simulink model "sampleModel27"  (R2021a)
settings: Solver=VariableStepAuto  StartTime=0.0  StopTime=10.0  RelTol=1e-3
undefined symbols (not defined in the file): DiscIntNeverNeededParam, magnitude, Newton, Raphson
libraries: simulink x49, pid_lib x7
(part 2 of 2)

== system sampleModel27/cfblk83/cfblk13/cfblk7 ==
  cfblk1 : Inport
  cfblk13 : Inport  Port=2
  cfblk10 : Constant  Value=[544016772.040966]  SampleTime=1
  cfblk11 : Constant  Value=[-953538141.984181]  SampleTime=1
  cfblk12 : Subsystem
  cfblk14 : Delay  SampleTime=1
  cfblk15 : Delay  SampleTime=1
  cfblk3 : simulink/Discrete/Transfer Fcn First Order  PoleZ=0.95  ICPrevOutput=0.0  DoSatur=off
  cfblk4 : DiscreteZeroPole  Poles=[0 0.5]  Gain=1
  cfblk5 : Sum  Inputs=|++
  cfblk6 : ComplexToMagnitudeAngle
  cfblk7 : Sum  Inputs=+
  cfblk8 : Polyval  Coefs=[ +2.081618890e-019, -1.441693666e-014, +4.719686976e-010, -8.536869453e-006, +1.621573104e-001, -8.087801117e+001 ]
  cfblk9 : UnaryMinus
  cfblk2 : Outport
  wires:
  cfblk6/1 -> cfblk8/1
  cfblk1/1 -> cfblk7/1
  cfblk13/1 -> cfblk6/1
  cfblk7/1 -> cfblk5/1
  cfblk10/1 -> cfblk2/1
  cfblk6/2 -> cfblk5/2
  cfblk8/1 -> cfblk4/1
  cfblk11/1 -> cfblk12/2(cfblk13)
  cfblk5/1 -> cfblk12/3(cfblk14)
  cfblk4/1 -> cfblk12/4(cfblk15)
  cfblk12/1(cfblk2) -> cfblk9/1
  cfblk12/2(cfblk17) -> cfblk3/1
  cfblk9/1 -> cfblk14/1
  cfblk14/1 -> cfblk12/5(cfblk16)
  cfblk3/1 -> cfblk15/1
  cfblk15/1 -> cfblk12/1(cfblk1)

== system sampleModel27/cfblk83/cfblk15/cfblk14 ==
  cfblk1 : Inport
  cfblk11 : Subsystem  TreatAsAtomicUnit=on
  cfblk12 : Subsystem  TreatAsAtomicUnit=on
  cfblk13 : Subsystem  TreatAsAtomicUnit=on
  cfblk14 : Subsystem  TreatAsAtomicUnit=on
  cfblk15 : Delay
  cfblk16 : Delay
  cfblk17 : Delay
  cfblk3 : UnitDelay  SampleTime=-1  HasFrameUpgradeWarning=on
  cfblk4 : Rounding
  cfblk5 : Constant  Value=[-440599559.077869]  SampleTime=1
  cfblk6 : Constant  Value=[542136050.953861]  SampleTime=1
  cfblk7 : Constant  Value=[-811490102.664521]  SampleTime=1
  cfblk8 : If  IfExpression=u1 >= 0  SampleTime=1
  cfblk9 : If  IfExpression=u1 >= 0  SampleTime=1
  cfblk2 : Outport
  cfblk10 : Outport  Port=2
  wires:
  cfblk1/1 -> cfblk14/1(cfblk1)
  cfblk6/1 -> cfblk2/1, cfblk8/1
  cfblk14/1(cfblk2) -> cfblk4/1, cfblk11/4(cfblk16), cfblk11/5(cfblk17), cfblk12/6(cfblk15)
  cfblk12/1(cfblk2) -> cfblk10/1
  cfblk5/1 -> cfblk3/1, cfblk12/3(cfblk12), cfblk12/5(cfblk14)
  cfblk7/1 -> cfblk14/2(cfblk16)
  cfblk4/1 -> cfblk11/3(cfblk15), cfblk15/1
  cfblk3/1 -> cfblk13/3(cfblk9), cfblk12/2(cfblk11), cfblk13/4(cfblk10), cfblk12/4(cfblk13)
  cfblk13/2(cfblk11) -> cfblk12/1(cfblk1)
  cfblk12/2(cfblk16) -> cfblk11/1(cfblk1)
  cfblk12/3(cfblk17) -> cfblk11/2(cfblk14)
  cfblk8/1 -> cfblk11/Action
  cfblk8/2 -> cfblk12/Action
  cfblk9/1 -> cfblk13/Action
  cfblk9/2 -> cfblk14/Action
  cfblk15/1 -> cfblk13/2(cfblk8)
  cfblk13/1(cfblk2) -> cfblk16/1
  cfblk16/1 -> cfblk9/1
  cfblk11/1(cfblk2) -> cfblk17/1
  cfblk17/1 -> cfblk13/1(cfblk1)

== system sampleModel27/cfblk83/cfblk15/cfblk15 ==
  cfblk1 : Inport
  cfblk9 : Inport  Port=2
  cfblk10 : Inport  Port=3
  cfblk3 : UnitDelay  SampleTime=-1  HasFrameUpgradeWarning=on
  cfblk4 : Abs
  cfblk5 : Bias  Bias=[477951449.519788]
  cfblk6 : Signum
  cfblk7 : Constant  Value=[-305255151.723231]  SampleTime=1
  cfblk8 : Subsystem
  cfblk2 : Outport
  wires:
  cfblk8/1(cfblk2) -> cfblk2/1
  cfblk1/1 -> cfblk5/1
  cfblk10/1 -> cfblk3/1
  cfblk3/1 -> cfblk6/1
  cfblk7/1 -> cfblk8/1(cfblk1)
  cfblk9/1 -> cfblk8/2(cfblk12)
  cfblk6/1 -> cfblk8/3(cfblk13)
  cfblk5/1 -> cfblk4/1
  cfblk4/1 -> cfblk8/4(cfblk14)

== system sampleModel27/cfblk83/cfblk16/cfblk13 ==
  cfblk1 : Inport
  cfblk7 : Inport  Port=2
  Action Port : ActionPort  ActionPortLabel=if(u1 >= 0)
  cfblk3 : simulink/Discrete/Transfer Fcn Lead or Lag  PoleZ=0.95  ZeroZ=0.75  ICPrevOutput=0.0  ICPrevInput=0.0  DoSatur=off
      settings: SourceProductBaseCode=SL
  cfblk4 : Bias  Bias=[-879373629.751207]
  cfblk5 : Constant  Value=[-106545189.607481]  SampleTime=1
  cfblk6 : Subsystem
  cfblk2 : Outport
  cfblk8 : Outport  Port=2
  wires:
  cfblk6/1(cfblk2) -> cfblk3/1
  cfblk3/1 -> cfblk2/1
  cfblk4/1 -> cfblk6/1(cfblk1)
  cfblk5/1 -> cfblk8/1, cfblk6/3(cfblk7)
  cfblk1/1 -> cfblk6/2(cfblk6)
  cfblk7/1 -> cfblk4/1

== system sampleModel27/cfblk83/cfblk16/cfblk14 ==
  cfblk1 : Inport
  cfblk8 : Inport  Port=2
  cfblk9 : Inport  Port=3
  cfblk10 : Inport  Port=4
  Action Port : ActionPort  ActionPortLabel=else
  cfblk3 : DiscreteFilter
  cfblk4 : Delay  ShowEnablePort=on
      settings: InputPortMap=u0,e6
  cfblk5 : Sqrt  Operator=rSqrt  AlgorithmType=Newton-Raphson  SaturateOnIntegerOverflow=on
  cfblk6 : Constant  Value=[-897019251.439010]  SampleTime=1
  cfblk7 : Constant  Value=[609715511.486789]  SampleTime=1
  cfblk2 : Outport
  cfblk11 : Outport  Port=2
  wires:
  cfblk7/1 -> cfblk2/1
  cfblk3/1 -> cfblk11/1
  cfblk8/1 -> cfblk5/1
  cfblk10/1 -> cfblk4/1
  cfblk1/1 -> cfblk3/1
  cfblk5/1 -> cfblk4/2

== system sampleModel27/cfblk84/cfblk8/cfblk14 ==
  cfblk1 : Inport
  cfblk11 : Inport  Port=2
  cfblk12 : Inport  Port=3
  Action Port : ActionPort  ActionPortLabel=if(u1 >= 0)
  cfblk10 : Constant  Value=[-145871612.215091]  SampleTime=1
  cfblk3 : Assignment  DiagnosticForDimensions=Warning  IndexOptions=Index vector (dialog)  Indices=1  OutputSizes=1
  cfblk4 : Sum  Inputs=|++
  cfblk5 : Sin  TimeSource=Use external signal  SampleTime=0
  cfblk6 : simulink/Math Operations/Slider Gain  gain=1  low=0  high=2
  cfblk7 : ComplexToRealImag
  cfblk8 : Constant  Value=[250736234.971967]  SampleTime=1
  cfblk9 : Constant  Value=[488356432.647786]  SampleTime=1
  cfblk2 : Outport
  cfblk13 : Outport  Port=2
  cfblk14 : Outport  Port=3
  wires:
  cfblk6/1 -> cfblk5/1
  cfblk9/1 -> cfblk13/1
  cfblk10/1 -> cfblk6/1
  cfblk8/1 -> cfblk2/1
  cfblk5/1 -> cfblk7/1
  cfblk3/1 -> cfblk14/1
  cfblk1/1 -> cfblk4/1
  cfblk11/1 -> cfblk3/1
  cfblk7/1 -> cfblk3/2
  cfblk7/2 -> cfblk4/2

== system sampleModel27/cfblk84/cfblk8/cfblk15 ==
  cfblk1 : Inport
  Action Port : ActionPort  ActionPortLabel=else
  cfblk3 : Bias  Bias=[98527291.273946]
  cfblk4 : Abs
  cfblk5 : Sqrt  Operator=rSqrt  AlgorithmType=Newton-Raphson  SaturateOnIntegerOverflow=on
  cfblk6 : Constant  Value=[946049467.563977]  SampleTime=1
  cfblk7 : Constant  Value=[-597347827.612500]  SampleTime=1
  cfblk8 : Constant  Value=[-404668651.330563]  SampleTime=1
  cfblk9 : Constant  Value=[83472011.768582]  SampleTime=1
  cfblk2 : Outport
  cfblk10 : Outport  Port=2
  cfblk11 : Outport  Port=3
  cfblk12 : Outport  Port=4
  wires:
  cfblk9/1 -> cfblk10/1
  cfblk1/1 -> cfblk2/1
  cfblk7/1 -> cfblk4/1
  cfblk5/1 -> cfblk3/1
  cfblk3/1 -> cfblk12/1
  cfblk8/1 -> cfblk5/1
  cfblk6/1 -> cfblk11/1

== system sampleModel27/cfblk85/cfblk13/cfblk10 ==
  cfblk1 : Inport
  cfblk10 : Inport  Port=2
  cfblk3 : DiscreteTransferFcn  SampleTime=1
  cfblk4 : Sum  Inputs=+
  cfblk5 : Gain  Gain=[765173450.202600]
  cfblk6 : Product  Inputs=*
  cfblk7 : Constant  Value=[-41618691.561886]  SampleTime=1
  cfblk8 : Constant  Value=[951977228.502192]  SampleTime=1
  cfblk9 : Constant  Value=[-841974024.752208]  SampleTime=1
  cfblk2 : Outport
  cfblk11 : Outport  Port=2
  cfblk12 : Outport  Port=3
  wires:
  cfblk9/1 -> cfblk3/1
  cfblk6/1 -> cfblk2/1
  cfblk8/1 -> cfblk4/1
  cfblk4/1 -> cfblk11/1
  cfblk5/1 -> cfblk12/1
  cfblk1/1 -> cfblk5/1
  cfblk7/1 -> cfblk6/1

== system sampleModel27/cfblk87/cfblk14/cfblk13 ==
  cfblk1 : Inport
  cfblk6 : Inport  Port=2
  cfblk7 : Inport  Port=3
  cfblk8 : Inport  Port=4
  cfblk3 : Sum  Inputs=+
  cfblk4 : MinMax  Inputs=3
  cfblk5 : Constant  Value=[-945013727.869418]  SampleTime=1
  cfblk2 : Outport
  cfblk9 : Outport  Port=2
  wires:
  cfblk7/1 -> cfblk4/1
  cfblk6/1 -> cfblk4/2
  cfblk5/1 -> cfblk3/1
  cfblk8/1 -> cfblk2/1
  cfblk1/1 -> cfblk9/1
  cfblk3/1 -> cfblk4/3

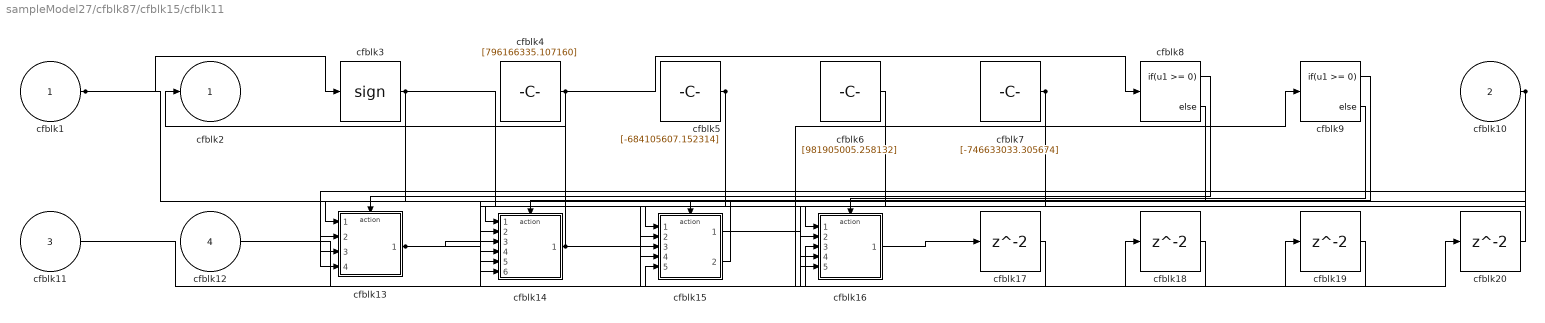
== system sampleModel27/cfblk87/cfblk15/cfblk11 ==
  cfblk1 : Inport
  cfblk10 : Inport  Port=2
  cfblk11 : Inport  Port=3
  cfblk12 : Inport  Port=4
  cfblk13 : Subsystem  TreatAsAtomicUnit=on
  cfblk14 : Subsystem  TreatAsAtomicUnit=on
  cfblk15 : Subsystem  TreatAsAtomicUnit=on
  cfblk16 : Subsystem  TreatAsAtomicUnit=on
  cfblk{17..20} (4 alike) : Delay
  cfblk3 : Signum
  cfblk4 : Constant  Value=[796166335.107160]  SampleTime=1
  cfblk5 : Constant  Value=[-684105607.152314]  SampleTime=1
  cfblk6 : Constant  Value=[981905005.258132]  SampleTime=1
  cfblk7 : Constant  Value=[-746633033.305674]  SampleTime=1
  cfblk8 : If  IfExpression=u1 >= 0  SampleTime=1
  cfblk9 : If  IfExpression=u1 >= 0  SampleTime=1
  cfblk2 : Outport
  wires:
  cfblk5/1 -> cfblk15/1(cfblk1), cfblk14/2(cfblk11)
  cfblk14/1(cfblk2) -> cfblk2/1, cfblk19/1, cfblk20/1
  cfblk10/1 -> cfblk16/1(cfblk1), cfblk13/4(cfblk10)
  cfblk1/1 -> cfblk3/1, cfblk14/5(cfblk14)
  cfblk11/1 -> cfblk9/1
  cfblk4/1 -> cfblk8/1, cfblk14/4(cfblk13)
  cfblk15/1(cfblk2) -> cfblk16/2(cfblk8)
  cfblk7/1 -> cfblk15/2(cfblk12), cfblk16/5(cfblk11), cfblk14/6(cfblk15)
  cfblk6/1 -> cfblk14/1(cfblk1)
  cfblk3/1 -> cfblk15/3(cfblk13), cfblk13/3(cfblk9)
  cfblk13/1(cfblk2) -> cfblk14/3(cfblk12), cfblk18/1
  cfblk15/2(cfblk16) -> cfblk13/1(cfblk1)
  cfblk12/1 -> cfblk16/3(cfblk9)
  cfblk8/1 -> cfblk13/Action
  cfblk8/2 -> cfblk14/Action
  cfblk9/1 -> cfblk15/Action
  cfblk9/2 -> cfblk16/Action
  cfblk16/1(cfblk2) -> cfblk17/1
  cfblk17/1 -> cfblk15/4(cfblk14)
  cfblk18/1 -> cfblk15/5(cfblk15)
  cfblk19/1 -> cfblk16/4(cfblk10)
  cfblk20/1 -> cfblk13/2(cfblk8)

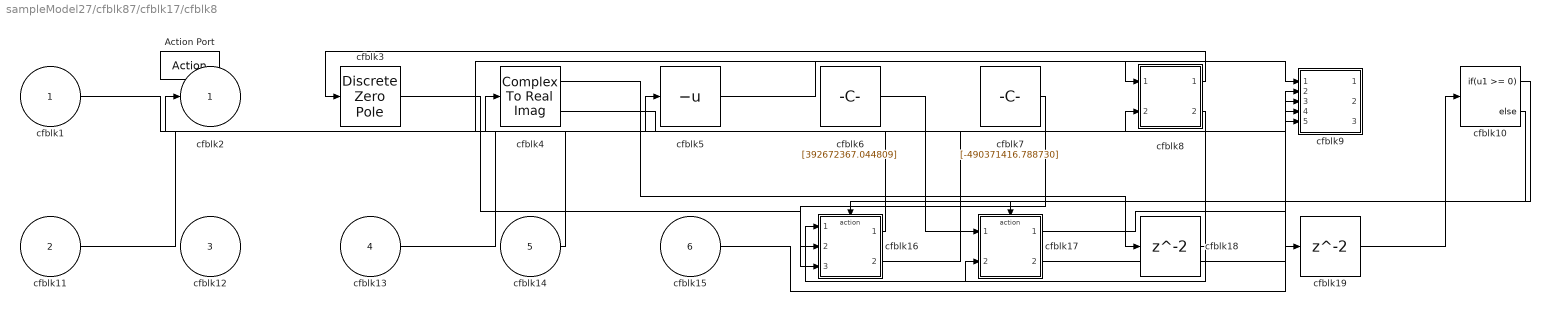
== system sampleModel27/cfblk87/cfblk17/cfblk8 ==
  cfblk1 : Inport
  cfblk11 : Inport  Port=2
  cfblk12 : Inport  Port=3
  cfblk13 : Inport  Port=4
  cfblk14 : Inport  Port=5
  cfblk15 : Inport  Port=6
  Action Port : ActionPort  ActionPortLabel=if(u1 >= 0)
  cfblk10 : If  IfExpression=u1 >= 0  SampleTime=1
  cfblk16 : Subsystem  TreatAsAtomicUnit=on
  cfblk17 : Subsystem  TreatAsAtomicUnit=on
  cfblk18 : Delay
  cfblk19 : Delay
  cfblk3 : DiscreteZeroPole  Poles=[0 0.5]  Gain=1  SampleTime=-1
  cfblk4 : ComplexToRealImag
  cfblk5 : UnaryMinus
  cfblk6 : Constant  Value=[392672367.044809]  SampleTime=1
  cfblk7 : Constant  Value=[-490371416.788730]  SampleTime=1
  cfblk8 : Subsystem
  cfblk9 : Subsystem
  cfblk2 : Outport
  wires:
  cfblk16/1(cfblk2) -> cfblk4/1
  cfblk11/1 -> cfblk8/1(cfblk1)
  cfblk8/1(cfblk2) -> cfblk3/1
  cfblk14/1 -> cfblk2/1
  cfblk6/1 -> cfblk17/1(cfblk1)
  cfblk13/1 -> cfblk5/1
  cfblk8/2(cfblk11) -> cfblk16/1(cfblk1)
  cfblk1/1 -> cfblk8/2(cfblk10)
  cfblk5/1 -> cfblk9/1(cfblk1)
  cfblk7/1 -> cfblk16/2(cfblk10)
  cfblk15/1 -> cfblk9/2(cfblk8)
  cfblk3/1 -> cfblk16/3(cfblk11)
  cfblk4/2 -> cfblk9/3(cfblk9)
  cfblk16/2(cfblk12) -> cfblk9/4(cfblk10)
  cfblk17/2(cfblk7) -> cfblk9/5(cfblk11)
  cfblk10/1 -> cfblk16/Action
  cfblk10/2 -> cfblk17/Action
  cfblk4/1 -> cfblk18/1
  cfblk18/1 -> cfblk17/2(cfblk6)
  cfblk17/1(cfblk2) -> cfblk19/1
  cfblk19/1 -> cfblk10/1

== system sampleModel27/cfblk87/cfblk17/cfblk9 ==
  cfblk1 : Inport
  cfblk11 : Inport  Port=2
  cfblk12 : Inport  Port=3
  cfblk13 : Inport  Port=4
  Action Port : ActionPort  ActionPortLabel=else
  cfblk10 : Subsystem
  cfblk14 : Delay
  cfblk3 : UnitDelay  SampleTime=-1  HasFrameUpgradeWarning=on
  cfblk4 : Assignment  DiagnosticForDimensions=Warning  IndexOptions=Index vector (dialog)  Indices=1  OutputSizes=1
  cfblk5 : Reshape
  cfblk6 : Constant  Value=[465556095.610833]  SampleTime=1
  cfblk7 : Constant  Value=[-882674569.855004]  SampleTime=1
  cfblk8 : Constant  Value=[-820974343.332864]  SampleTime=1
  cfblk9 : Constant  Value=[896340327.104104]  SampleTime=1
  cfblk2 : Outport
  wires:
  cfblk5/1 -> cfblk4/1
  cfblk10/1(cfblk2) -> cfblk4/2
  cfblk7/1 -> cfblk10/1(cfblk1)
  cfblk1/1 -> cfblk2/1
  cfblk3/1 -> cfblk5/1
  cfblk9/1 -> cfblk10/2(cfblk8)
  cfblk8/1 -> cfblk10/3(cfblk9)
  cfblk11/1 -> cfblk10/4(cfblk10)
  cfblk4/1 -> cfblk14/1
  cfblk14/1 -> cfblk3/1

== system sampleModel27/cfblk88/cfblk11/cfblk6 ==
  cfblk1 : Inport
  cfblk11 : Inport  Port=2
  cfblk12 : Inport  Port=3
  cfblk10 : Constant  Value=[780851204.861315]  SampleTime=1
  cfblk13 : Delay
  cfblk3 : UnitDelay  SampleTime=-1  HasFrameUpgradeWarning=on
  cfblk4 : simulink/Discrete/Difference  ICPrevInput=0.0  OutMin=[]  OutMax=[]  OutDataTypeStr=Inherit: Inherit via back propagation  OutDataType=fixdt(1, 16)  OutScaling=2^-10  DoSatur=off
  cfblk5 : PermuteDimensions
  cfblk6 : Sum  Inputs=+
  cfblk7 : Squeeze
  cfblk8 : Signum
  cfblk9 : Polyval  Coefs=[ +2.081618890e-019, -1.441693666e-014, +4.719686976e-010, -8.536869453e-006, +1.621573104e-001, -8.087801117e+001 ]
  cfblk2 : Outport
  wires:
  cfblk1/1 -> cfblk3/1
  cfblk10/1 -> cfblk9/1
  cfblk8/1 -> cfblk4/1
  cfblk3/1 -> cfblk8/1
  cfblk9/1 -> cfblk2/1
  cfblk12/1 -> cfblk6/1
  cfblk5/1 -> cfblk7/1
  cfblk7/1 -> cfblk13/1
  cfblk13/1 -> cfblk5/1

== system sampleModel27/cfblk93/cfblk11/cfblk14 ==
  cfblk1 : Inport
  cfblk9 : Inport  Port=2
  cfblk10 : Inport  Port=3
  cfblk11 : Delay
  cfblk3 : DiscreteIntegrator  SampleTime=-1  ICPrevOutput=DiscIntNeverNeededParam  ICPrevScaledInput=DiscIntNeverNeededParam
  cfblk4 : simulink/Discrete/Transfer Fcn First Order  PoleZ=0.95  ICPrevOutput=0.0  DoSatur=off
  cfblk5 : Signum
  cfblk6 : Constant  Value=[-675553357.421443]  SampleTime=1
  cfblk7 : Constant  Value=[-161102993.880450]  SampleTime=1
  cfblk8 : Subsystem
  cfblk2 : Outport
  wires:
  cfblk8/1(cfblk2) -> cfblk3/1
  cfblk5/1 -> cfblk4/1
  cfblk1/1 -> cfblk5/1
  cfblk10/1 -> cfblk2/1
  cfblk7/1 -> cfblk8/2(cfblk6)
  cfblk6/1 -> cfblk8/3(cfblk7)
  cfblk9/1 -> cfblk8/4(cfblk8)
  cfblk4/1 -> cfblk8/5(cfblk9)
  cfblk3/1 -> cfblk11/1
  cfblk11/1 -> cfblk8/1(cfblk1)

== system sampleModel27/cfblk93/cfblk11/cfblk18 ==
  cfblk1 : Inport
  cfblk11 : Inport  Port=2
  Action Port : ActionPort  ActionPortLabel=if(u1 >= 0)
  cfblk10 : Subsystem
  cfblk13 : Delay
  cfblk14 : Delay
  cfblk15 : Delay
  cfblk3 : simulink/Discrete/Difference  ICPrevInput=0.0  OutMin=[]  OutMax=[]  OutDataTypeStr=Inherit: Inherit via back propagation  OutDataType=fixdt(1, 16)  OutScaling=2^-10  DoSatur=off
  cfblk4 : Sin  TimeSource=Use external signal  SampleTime=0
  cfblk5 : Math  Operator=mod  SaturateOnIntegerOverflow=on
  cfblk6 : ComplexToMagnitudeAngle
  cfblk7 : Polyval  Coefs=[ +2.081618890e-019, -1.441693666e-014, +4.719686976e-010, -8.536869453e-006, +1.621573104e-001, -8.087801117e+001 ]
  cfblk8 : simulink/Math Operations/Slider Gain  gain=1  low=0  high=2
  cfblk9 : Constant  Value=[-165486914.707438]  SampleTime=1
  cfblk2 : Outport
  cfblk12 : Outport  Port=2
  wires:
  cfblk6/1 -> cfblk3/1
  cfblk1/1 -> cfblk2/1, cfblk10/6(cfblk12)
  cfblk8/1 -> cfblk4/1
  cfblk10/1(cfblk2) -> cfblk6/1, cfblk12/1
  cfblk7/1 -> cfblk8/1, cfblk14/1
  cfblk4/1 -> cfblk5/1
  cfblk11/1 -> cfblk10/1(cfblk1), cfblk5/2
  cfblk9/1 -> cfblk10/2(cfblk8)
  cfblk3/1 -> cfblk7/1
  cfblk5/1 -> cfblk13/1
  cfblk13/1 -> cfblk10/3(cfblk9)
  cfblk14/1 -> cfblk10/5(cfblk11)
  cfblk6/2 -> cfblk15/1
  cfblk15/1 -> cfblk10/4(cfblk10)

== system sampleModel27/cfblk93/cfblk11/cfblk19 ==
  cfblk1 : Inport
  cfblk9 : Inport  Port=2
  Action Port : ActionPort  ActionPortLabel=else
  cfblk11 : Delay
  cfblk3 : simulink/Discrete/Transfer Fcn Lead or Lag  PoleZ=0.95  ZeroZ=0.75  ICPrevOutput=0.0  ICPrevInput=0.0  DoSatur=off
      settings: SourceProductBaseCode=SL
  cfblk4 : Gain  Gain=[803756219.066566]
  cfblk5 : Constant  Value=[818842009.300380]  SampleTime=1
  cfblk6 : Constant  Value=[505307302.116209]  SampleTime=1
  cfblk7 : Constant  Value=[166707104.020552]  SampleTime=1
  cfblk8 : Subsystem
  cfblk2 : Outport
  cfblk10 : Outport  Port=2
  wires:
  cfblk8/1(cfblk2) -> cfblk4/1
  cfblk8/2(cfblk8) -> cfblk10/1
  cfblk1/1 -> cfblk2/1
  cfblk6/1 -> cfblk3/1
  cfblk3/1 -> cfblk8/2(cfblk7)
  cfblk4/1 -> cfblk11/1
  cfblk11/1 -> cfblk8/1(cfblk1)

== system sampleModel27/cfblk93/cfblk12/cfblk6 ==
  cfblk1 : Inport
  cfblk6 : Inport  Port=2
  cfblk3 : DiscreteIntegrator  SampleTime=-1  ICPrevOutput=DiscIntNeverNeededParam  ICPrevScaledInput=DiscIntNeverNeededParam
  cfblk4 : Sum  Inputs=+
  cfblk5 : Constant  Value=[149687148.912851]  SampleTime=1
  cfblk2 : Outport
  cfblk7 : Outport  Port=2
  wires:
  cfblk4/1 -> cfblk2/1
  cfblk5/1 -> cfblk4/1
  cfblk6/1 -> cfblk7/1
  cfblk1/1 -> cfblk3/1

== system sampleModel27/cfblk95/cfblk12/cfblk10 ==
  cfblk1 : Inport
  cfblk7 : Inport  Port=2
  cfblk8 : Inport  Port=3
  Action Port : ActionPort  ActionPortLabel=if(u1 >= 0)
  cfblk3 : Delay  DelayLengthSource=Input port
      settings: InputPortMap=u0,p1
  cfblk4 : Delay
  cfblk5 : Sum  Inputs=+
  cfblk6 : DotProduct  InputSameDT=on  OutDataTypeStr=Inherit: Inherit via internal rule
  cfblk2 : Outport
  wires:
  cfblk6/1 -> cfblk3/1
  cfblk5/1 -> cfblk6/1
  cfblk8/1 -> cfblk3/2
  cfblk1/1 -> cfblk4/1
  cfblk3/1 -> cfblk2/1
  cfblk7/1 -> cfblk6/2
  cfblk4/1 -> cfblk5/1

== system sampleModel27/cfblk95/cfblk12/cfblk11 ==
  cfblk1 : Inport
  cfblk12 : Inport  Port=2
  cfblk13 : Inport  Port=3
  cfblk14 : Inport  Port=4
  cfblk15 : Inport  Port=5
  Action Port : ActionPort  ActionPortLabel=else
  cfblk10 : Subsystem
  cfblk11 : Subsystem
  cfblk3 : simulink/Discrete/Transfer Fcn First Order  PoleZ=0.95  ICPrevOutput=0.0  DoSatur=off
  cfblk4 : ComplexToRealImag
  cfblk5 : UnaryMinus
  cfblk6 : Constant  Value=[-499085242.561291]  SampleTime=1
  cfblk7 : Constant  Value=[891439870.689055]  SampleTime=1
  cfblk8 : Constant  Value=[-658449447.398283]  SampleTime=1
  cfblk9 : Constant  Value=[112371694.330315]  SampleTime=1
  cfblk2 : Outport
  cfblk16 : Outport  Port=2
  wires:
  cfblk9/1 -> cfblk5/1
  cfblk14/1 -> cfblk11/1(cfblk1)
  cfblk13/1 -> cfblk10/1(cfblk1)
  cfblk1/1 -> cfblk11/2(cfblk16)
  cfblk8/1 -> cfblk4/1
  cfblk3/1 -> cfblk10/2(cfblk8)
  cfblk10/1(cfblk2) -> cfblk2/1
  cfblk12/1 -> cfblk16/1
  cfblk15/1 -> cfblk10/3(cfblk9)
  cfblk6/1 -> cfblk10/4(cfblk10)
  cfblk7/1 -> cfblk3/1

== system sampleModel27/cfblk83/cfblk13/cfblk7/cfblk12 ==
  cfblk1 : Inport
  cfblk13 : Inport  Port=2
  cfblk14 : Inport  Port=3
  cfblk15 : Inport  Port=4
  cfblk16 : Inport  Port=5
  cfblk10 : Constant  Value=[-268449300.692861]  SampleTime=1
  cfblk11 : Constant  Value=[-358015095.302553]  SampleTime=1
  cfblk12 : Constant  Value=[-762579594.381282]  SampleTime=1
  cfblk3 : UnitDelay  HasFrameUpgradeWarning=on
  cfblk4 : Product  Inputs=*
  cfblk5 : Product  Inputs=**
  cfblk6 : PermuteDimensions
  cfblk7 : simulink/Math Operations/MinMax Running Resettable  Function=min  vinit=0.0
  cfblk8 : Product  Inputs=*
  cfblk9 : Constant  Value=[954786102.000246]  SampleTime=1
  cfblk2 : Outport
  cfblk17 : Outport  Port=2
  wires:
  cfblk14/1 -> cfblk17/1
  cfblk6/1 -> cfblk7/1
  cfblk4/1 -> cfblk8/1
  cfblk5/1 -> cfblk3/1
  cfblk12/1 -> cfblk5/1
  cfblk16/1 -> cfblk4/1
  cfblk1/1 -> cfblk6/1
  cfblk3/1 -> cfblk7/2
  cfblk10/1 -> cfblk5/2
  cfblk11/1 -> cfblk2/1

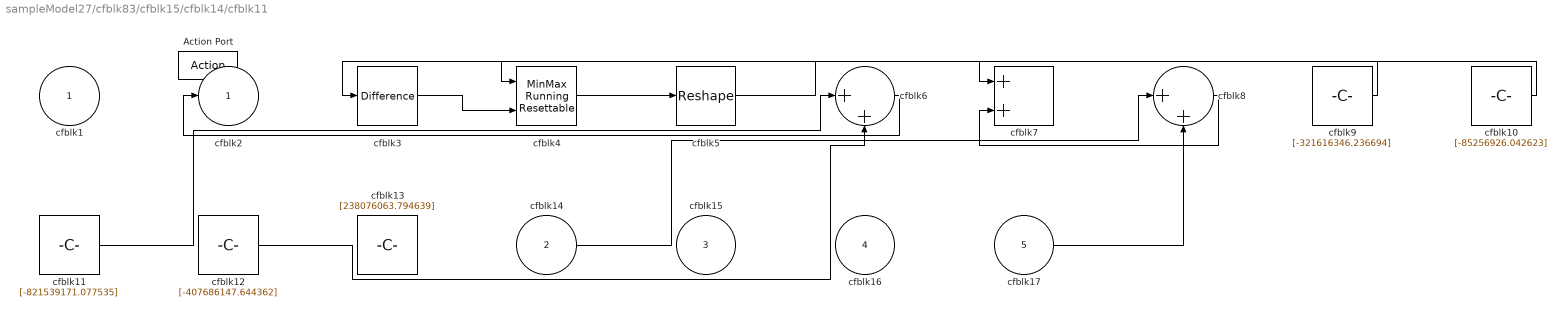
== system sampleModel27/cfblk83/cfblk15/cfblk14/cfblk11 ==
  cfblk1 : Inport
  cfblk14 : Inport  Port=2
  cfblk15 : Inport  Port=3
  cfblk16 : Inport  Port=4
  cfblk17 : Inport  Port=5
  Action Port : ActionPort  ActionPortLabel=if(u1 >= 0)
  cfblk10 : Constant  Value=[-85256926.042623]  SampleTime=1
  cfblk11 : Constant  Value=[-821539171.077535]  SampleTime=1
  cfblk12 : Constant  Value=[-407686147.644362]  SampleTime=1
  cfblk13 : Constant  Value=[238076063.794639]  SampleTime=1
  cfblk3 : simulink/Discrete/Difference  ICPrevInput=0.0  OutMin=[]  OutMax=[]  OutDataTypeStr=Inherit: Inherit via back propagation  OutDataType=fixdt(1, 16)  OutScaling=2^-10  DoSatur=off
  cfblk4 : simulink/Math Operations/MinMax Running Resettable  Function=min  vinit=0.0
  cfblk5 : Reshape
  cfblk6 : Sum  Inputs=|++
  cfblk7 : Sum
  cfblk8 : Sum  Inputs=|++
  cfblk9 : Constant  Value=[-321616346.236694]  SampleTime=1
  cfblk2 : Outport
  wires:
  cfblk11/1 -> cfblk6/1
  cfblk10/1 -> cfblk3/1
  cfblk5/1 -> cfblk7/1
  cfblk14/1 -> cfblk8/1
  cfblk6/1 -> cfblk2/1
  cfblk12/1 -> cfblk6/2
  cfblk4/1 -> cfblk5/1
  cfblk9/1 -> cfblk4/1
  cfblk3/1 -> cfblk4/2
  cfblk17/1 -> cfblk8/2
  cfblk8/1 -> cfblk7/2

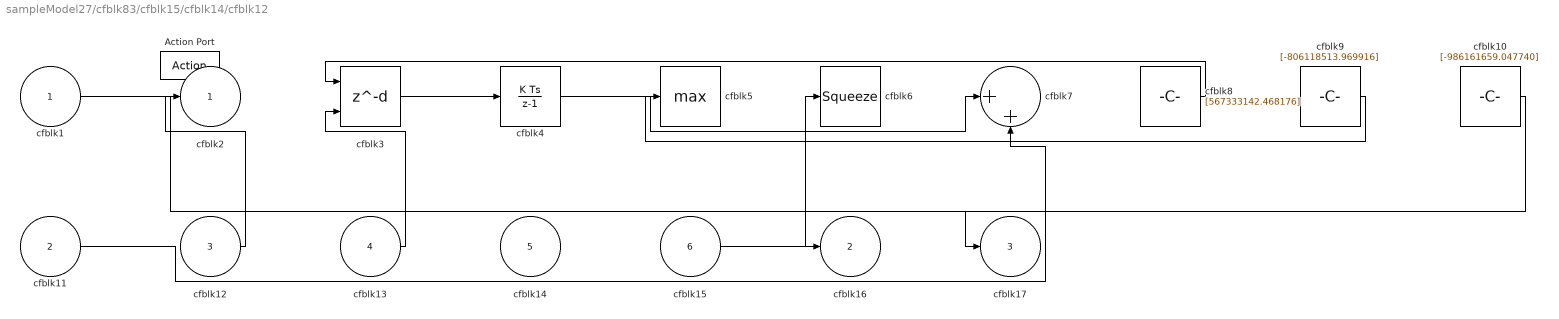
== system sampleModel27/cfblk83/cfblk15/cfblk14/cfblk12 ==
  cfblk1 : Inport
  cfblk11 : Inport  Port=2
  cfblk12 : Inport  Port=3
  cfblk13 : Inport  Port=4
  cfblk14 : Inport  Port=5
  cfblk15 : Inport  Port=6
  Action Port : ActionPort  ActionPortLabel=else
  cfblk10 : Constant  Value=[-986161659.047740]  SampleTime=1
  cfblk3 : Delay  DelayLengthSource=Input port
      settings: InputPortMap=u0,p1
  cfblk4 : DiscreteIntegrator  SampleTime=-1  ICPrevOutput=DiscIntNeverNeededParam  ICPrevScaledInput=DiscIntNeverNeededParam
  cfblk5 : MinMax  Function=max
  cfblk6 : Squeeze
  cfblk7 : Sum  Inputs=|++
  cfblk8 : Constant  Value=[567333142.468176]  SampleTime=1
  cfblk9 : Constant  Value=[-806118513.969916]  SampleTime=1
  cfblk2 : Outport
  cfblk16 : Outport  Port=2
  cfblk17 : Outport  Port=3
  wires:
  cfblk1/1 -> cfblk17/1
  cfblk8/1 -> cfblk3/1
  cfblk4/1 -> cfblk7/1
  cfblk13/1 -> cfblk3/2
  cfblk9/1 -> cfblk5/1
  cfblk11/1 -> cfblk7/2
  cfblk12/1 -> cfblk2/1
  cfblk3/1 -> cfblk4/1
  cfblk15/1 -> cfblk6/1
  cfblk10/1 -> cfblk16/1

== system sampleModel27/cfblk83/cfblk15/cfblk14/cfblk13 ==
  cfblk1 : Inport
  cfblk8 : Inport  Port=2
  cfblk9 : Inport  Port=3
  cfblk10 : Inport  Port=4
  Action Port : ActionPort  ActionPortLabel=if(u1 >= 0)
  cfblk3 : Trigonometry
  cfblk4 : Constant  Value=[-710237360.327621]  SampleTime=1
  cfblk5 : Constant  Value=[-76118424.905763]  SampleTime=1
  cfblk6 : Constant  Value=[-943105026.899090]  SampleTime=1
  cfblk7 : Constant  Value=[-867711988.809449]  SampleTime=1
  cfblk2 : Outport
  cfblk11 : Outport  Port=2
  wires:
  cfblk3/1 -> cfblk2/1
  cfblk6/1 -> cfblk3/1
  cfblk7/1 -> cfblk11/1

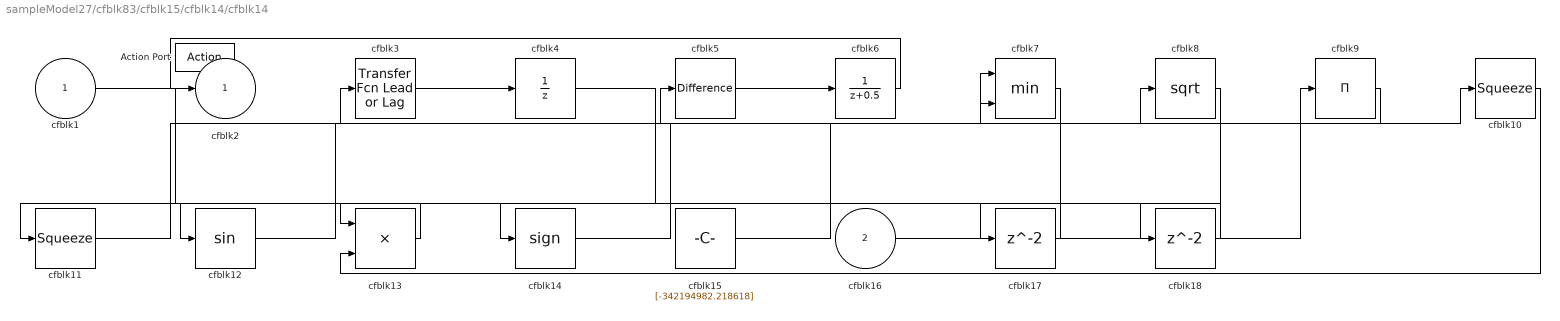
== system sampleModel27/cfblk83/cfblk15/cfblk14/cfblk14 ==
  cfblk1 : Inport
  cfblk16 : Inport  Port=2
  Action Port : ActionPort  ActionPortLabel=else
  cfblk10 : Squeeze
  cfblk11 : Squeeze
  cfblk12 : Trigonometry
  cfblk13 : Product  Inputs=**
  cfblk14 : Signum
  cfblk15 : Constant  Value=[-342194982.218618]  SampleTime=1
  cfblk17 : Delay
  cfblk18 : Delay
  cfblk3 : simulink/Discrete/Transfer Fcn Lead or Lag  PoleZ=0.95  ZeroZ=0.75  ICPrevOutput=0.0  ICPrevInput=0.0  DoSatur=off
      settings: SourceProductBaseCode=SL
  cfblk4 : UnitDelay  SampleTime=-1  HasFrameUpgradeWarning=on
  cfblk5 : simulink/Discrete/Difference  ICPrevInput=0.0  OutMin=[]  OutMax=[]  OutDataTypeStr=Inherit: Inherit via back propagation  OutDataType=fixdt(1, 16)  OutScaling=2^-10  DoSatur=off
  cfblk6 : DiscreteTransferFcn
  cfblk7 : MinMax  Inputs=2
  cfblk8 : Sqrt  SaturateOnIntegerOverflow=on
  cfblk9 : Product  Inputs=*
  cfblk2 : Outport
  wires:
  cfblk16/1 -> cfblk9/1
  cfblk8/1 -> cfblk12/1
  cfblk11/1 -> cfblk7/1
  cfblk5/1 -> cfblk6/1
  cfblk10/1 -> cfblk13/2
  cfblk13/1 -> cfblk11/1
  cfblk9/1 -> cfblk7/2
  cfblk3/1 -> cfblk4/1
  cfblk6/1 -> cfblk2/1
  cfblk14/1 -> cfblk10/1
  cfblk1/1 -> cfblk14/1
  cfblk15/1 -> cfblk8/1
  cfblk12/1 -> cfblk5/1
  cfblk7/1 -> cfblk17/1
  cfblk17/1 -> cfblk13/1
  cfblk4/1 -> cfblk18/1
  cfblk18/1 -> cfblk3/1

== system sampleModel27/cfblk83/cfblk15/cfblk15/cfblk8 ==
  cfblk1 : Inport
  cfblk12 : Inport  Port=2
  cfblk13 : Inport  Port=3
  cfblk14 : Inport  Port=4
  cfblk10 : ComplexToMagnitudeAngle
  cfblk11 : Constant  Value=[-383136241.761848]  SampleTime=1
  cfblk3 : Delay  DelayLengthSource=Input port
      settings: InputPortMap=u0,p1
  cfblk4 : simulink/Discrete/Difference  ICPrevInput=0.0  OutMin=[]  OutMax=[]  OutDataTypeStr=Inherit: Inherit via back propagation  OutDataType=fixdt(1, 16)  OutScaling=2^-10  DoSatur=off
  cfblk5 : DiscreteZeroPole  Poles=[0 0.5]  Gain=1  SampleTime=-1
  cfblk6 : Sqrt  Operator=rSqrt  AlgorithmType=Newton-Raphson  SaturateOnIntegerOverflow=on
  cfblk7 : UnaryMinus
  cfblk8 : Bias  Bias=[54533641.550614]
  cfblk9 : Rounding
  cfblk2 : Outport
  wires:
  cfblk1/1 -> cfblk8/1
  cfblk14/1 -> cfblk5/1
  cfblk8/1 -> cfblk2/1
  cfblk3/1 -> cfblk6/1
  cfblk9/1 -> cfblk3/1
  cfblk7/1 -> cfblk9/1
  cfblk4/1 -> cfblk3/2
  cfblk12/1 -> cfblk7/1
  cfblk5/1 -> cfblk10/1
  cfblk11/1 -> cfblk4/1

== system sampleModel27/cfblk83/cfblk16/cfblk13/cfblk6 ==
  cfblk1 : Inport
  cfblk6 : Inport  Port=2
  cfblk7 : Inport  Port=3
  cfblk3 : DiscreteZeroPole  Poles=[0 0.5]  Gain=1  SampleTime=-1
  cfblk4 : Product
  cfblk5 : ComplexToMagnitudeAngle
  cfblk8 : Delay
  cfblk2 : Outport
  wires:
  cfblk5/1 -> cfblk4/1
  cfblk7/1 -> cfblk2/1
  cfblk6/1 -> cfblk4/2
  cfblk3/1 -> cfblk5/1
  cfblk4/1 -> cfblk8/1
  cfblk8/1 -> cfblk3/1

== system sampleModel27/cfblk87/cfblk15/cfblk11/cfblk13 ==
  cfblk1 : Inport
  cfblk8 : Inport  Port=2
  cfblk9 : Inport  Port=3
  cfblk10 : Inport  Port=4
  Action Port : ActionPort  ActionPortLabel=if(u1 >= 0)
  cfblk3 : Product  Inputs=**
  cfblk4 : Squeeze
  cfblk5 : Signum
  cfblk6 : Constant  Value=[-934890208.211191]  SampleTime=1
  cfblk7 : Constant  Value=[739841428.666680]  SampleTime=1
  cfblk2 : Outport
  wires:
  cfblk6/1 -> cfblk3/1
  cfblk4/1 -> cfblk5/1
  cfblk5/1 -> cfblk2/1
  cfblk10/1 -> cfblk3/2
  cfblk1/1 -> cfblk4/1

== system sampleModel27/cfblk87/cfblk15/cfblk11/cfblk14 ==
  cfblk1 : Inport
  cfblk11 : Inport  Port=2
  cfblk12 : Inport  Port=3
  cfblk13 : Inport  Port=4
  cfblk14 : Inport  Port=5
  cfblk15 : Inport  Port=6
  Action Port : ActionPort  ActionPortLabel=else
  cfblk10 : Constant  Value=[679871546.871065]  SampleTime=1
  cfblk16 : Delay
  cfblk3 : simulink/Discrete/Transfer Fcn Lead or Lag  PoleZ=0.95  ZeroZ=0.75  ICPrevOutput=0.0  ICPrevInput=0.0  DoSatur=off
      settings: SourceProductBaseCode=SL
  cfblk4 : pid_lib/PID Controller  Controller=PID  Form=Parallel  TimeDomain=Discrete-time  UseExternalTs=off  SampleTime=-1  IntegratorMethod=Forward Euler  FilterMethod=Forward Euler  ControllerParametersSource=internal  P=1  I=1  D=0  UseFilter=on  N=100  TunerSelectOption=Transfer Function Based (PID Tuner App)  InitialConditionSource=internal  InitialConditionForIntegrator=0  InitialConditionForFilter=0  DifferentiatorICPrevScaledInput=0  ExternalReset=none  TrackingMode=off  Kt=1  LimitOutput=off  SatLimitsSource=internal  UpperSaturationLimit=inf  LowerSaturationLimit=-inf  LinearizeAsGain=off  AntiWindupMode=none  Kb=1  POutMin=[]  POutMax=[]  IOutMin=[]  IOutMax=[]  DOutMin=[]  DOutMax=[]  NOutMin=[]  NOutMax=[]  SumOutMin=[]  SumOutMax=[]  SaturationOutMin=[]  SaturationOutMax=[]  PParamMin=[]  PParamMax=[]  IParamMin=[]  IParamMax=[]  DParamMin=[]  DParamMax=[]  NParamMin=[]  NParamMax=[]  KbParamMin=[]  KbParamMax=[]  KtParamMin=[]  KtParamMax=[]  KbOutMin=[]  KbOutMax=[]  KtOutMin=[]  KtOutMax=[]  IntegratorOutMin=[]  IntegratorOutMax=[]  FilterOutMin=[]  FilterOutMax=[]  SumI1OutMin=[]  SumI1OutMax=[]  SumI2OutMin=[]  SumI2OutMax=[]  SumI3OutMin=[]  SumI3OutMax=[]  SumI4OutMin=[]  SumI4OutMax=[]  SumDOutMin=[]  SumDOutMax=[]  DifferentiatorOutMin=[]  DifferentiatorOutMax=[]  FilterDiffOutCoefMin=[]  FilterDiffOutCoefMax=[]  ReciprocalOutMin=[]  ReciprocalOutMax=[]  SumDenOutMin=[]  SumDenOutMax=[]  SumNumOutMin=[]  SumNumOutMax=[]  DivideOutMin=[]  DivideOutMax=[]  UdiffTsProdOutMin=[]  UdiffTsProdOutMax=[]  NTsProdOutMin=[]  NTsProdOutMax=[]  UintegralTsProdOutMin=[]  UintegralTsProdOutMax=[]  UngainTsProdOutMin=[]  UngainTsProdOutMax=[]  IntegratorContinuousStateAttributes=''  IntegratorStateMustResolveToSignalObject=off  IntegratorRTWStateStorageClass=Auto  FilterContinuousStateAttributes=''  FilterStateMustResolveToSignalObject=off  FilterRTWStateStorageClass=Auto  ParallelPVariant=InternalParameters  IdealPVariant=Disabled  IVariant=InternalParameters  DVariant=InternalParameters  IntegratorVariant=Discrete  SatVariant=Disabled  AWVariant=Passthrough  PCopyVariant=Disabled  TRVariant=Disabled  FdbkBlocksVariant=Forward  IdealPFdbkVariant=Disabled  SatFdbkVariant=Disabled  DerivativeFilterVariant=ForwardEulerFilter  NVariant=InternalParameters  NCopyVariant=Disabled  FilterICVariant=InternalICsFilter  IntegratorICVariant=InternalICs  ExternalResetVariant=Disabled  TRSumVariant=Passthrough  SumFdbkVariant=Disabled  SumVariant=Sum_PID  TsampFilterVariant=InternalTs  TsampNgainVariant=Passthrough  TsampIntegralVariant=Passthrough  ExternalSaturationOutDataTypeStr=Inherit: Same as second input
  cfblk5 : DiscreteIntegrator  SampleTime=-1  ICPrevOutput=DiscIntNeverNeededParam  ICPrevScaledInput=DiscIntNeverNeededParam
  cfblk6 : MinMax  Function=max  Inputs=3
  cfblk7 : Product
  cfblk8 : PermuteDimensions
  cfblk9 : Constant  Value=[-521457814.829251]  SampleTime=1
  cfblk2 : Outport
  wires:
  cfblk10/1 -> cfblk5/1
  cfblk15/1 -> cfblk4/1
  cfblk1/1 -> cfblk2/1
  cfblk9/1 -> cfblk8/1
  cfblk5/1 -> cfblk7/1
  cfblk7/1 -> cfblk6/1
  cfblk11/1 -> cfblk7/2
  cfblk3/1 -> cfblk6/2
  cfblk14/1 -> cfblk6/3
  cfblk6/1 -> cfblk16/1
  cfblk16/1 -> cfblk3/1

== system sampleModel27/cfblk87/cfblk15/cfblk11/cfblk15 ==
  cfblk1 : Inport
  cfblk12 : Inport  Port=2
  cfblk13 : Inport  Port=3
  cfblk14 : Inport  Port=4
  cfblk15 : Inport  Port=5
  Action Port : ActionPort  ActionPortLabel=if(u1 >= 0)
  cfblk10 : Constant  Value=[-331630096.819083]  SampleTime=1
  cfblk11 : Constant  Value=[-535526653.304140]  SampleTime=1
  cfblk3 : DiscreteTransferFcn
  cfblk4 : Signum
  cfblk5 : Sum  Inputs=+-
  cfblk6 : PermuteDimensions
  cfblk7 : Constant  Value=[374771752.374591]  SampleTime=1
  cfblk8 : Constant  Value=[103566890.028713]  SampleTime=1
  cfblk9 : Constant  Value=[956632047.868507]  SampleTime=1
  cfblk2 : Outport
  cfblk16 : Outport  Port=2
  wires:
  cfblk1/1 -> cfblk6/1
  cfblk14/1 -> cfblk5/1
  cfblk8/1 -> cfblk5/2
  cfblk5/1 -> cfblk16/1
  cfblk12/1 -> cfblk3/1
  cfblk7/1 -> cfblk2/1
  cfblk10/1 -> cfblk4/1

== system sampleModel27/cfblk87/cfblk15/cfblk11/cfblk16 ==
  cfblk1 : Inport
  cfblk8 : Inport  Port=2
  cfblk9 : Inport  Port=3
  cfblk10 : Inport  Port=4
  cfblk11 : Inport  Port=5
  Action Port : ActionPort  ActionPortLabel=else
  cfblk3 : Constant  Value=[-145636971.830146]  SampleTime=1
  cfblk4 : Constant  Value=[39399430.821719]  SampleTime=1
  cfblk5 : Constant  Value=[-228185624.455977]  SampleTime=1
  cfblk6 : Constant  Value=[4919590.459695]  SampleTime=1
  cfblk7 : Constant  Value=[-248548614.614052]  SampleTime=1
  cfblk2 : Outport
  wires:
  cfblk10/1 -> cfblk2/1

== system sampleModel27/cfblk87/cfblk17/cfblk8/cfblk16 ==
  cfblk1 : Inport
  cfblk10 : Inport  Port=2
  cfblk11 : Inport  Port=3
  Action Port : ActionPort  ActionPortLabel=if(u1 >= 0)
  cfblk13 : Delay
  cfblk3 : simulink/Discrete/Transfer Fcn Real Zero  ZeroZ=0.75  ICPrevInput=0.0  DoSatur=off
      settings: SourceProductBaseCode=SL
  cfblk4 : Sin  TimeSource=Use external signal  SampleTime=0
  cfblk5 : Abs
  cfblk6 : Polyval  Coefs=[ +2.081618890e-019, -1.441693666e-014, +4.719686976e-010, -8.536869453e-006, +1.621573104e-001, -8.087801117e+001 ]
  cfblk7 : simulink/Math Operations/MinMax Running Resettable  Function=min  vinit=0.0
  cfblk8 : Product
  cfblk9 : Constant  Value=[-222124711.616685]  SampleTime=1
  cfblk2 : Outport
  cfblk12 : Outport  Port=2
  wires:
  cfblk7/1 -> cfblk6/1
  cfblk11/1 -> cfblk12/1
  cfblk8/1 -> cfblk5/1
  cfblk4/1 -> cfblk2/1
  cfblk6/1 -> cfblk3/1
  cfblk9/1 -> cfblk4/1
  cfblk1/1 -> cfblk7/2
  cfblk3/1 -> cfblk8/1
  cfblk10/1 -> cfblk8/2
  cfblk5/1 -> cfblk13/1
  cfblk13/1 -> cfblk7/1

== system sampleModel27/cfblk87/cfblk17/cfblk8/cfblk17 ==
  cfblk1 : Inport
  cfblk6 : Inport  Port=2
  Action Port : ActionPort  ActionPortLabel=else
  cfblk3 : PermuteDimensions
  cfblk4 : Constant  Value=[-722766209.396215]  SampleTime=1
  cfblk5 : Constant  Value=[-732444055.707271]  SampleTime=1
  cfblk2 : Outport
  cfblk7 : Outport  Port=2
  wires:
  cfblk6/1 -> cfblk2/1
  cfblk4/1 -> cfblk3/1
  cfblk5/1 -> cfblk7/1

== system sampleModel27/cfblk87/cfblk17/cfblk8/cfblk8 ==
  cfblk1 : Inport
  cfblk10 : Inport  Port=2
  cfblk3 : simulink/Discrete/Tapped Delay  vinit=0.0  samptime=-1  NumDelays=1  DelayOrder=Oldest  includeCurrent=off
  cfblk4 : Sin  TimeSource=Use external signal  SampleTime=0
  cfblk5 : simulink/Math Operations/Slider Gain  gain=1  low=0  high=2
  cfblk6 : MinMax  Function=max  Inputs=2
  cfblk7 : Bias  Bias=[354819331.107694]
  cfblk8 : Constant  Value=[413709704.343942]  SampleTime=1
  cfblk9 : Constant  Value=[-922772328.033709]  SampleTime=1
  cfblk2 : Outport
  cfblk11 : Outport  Port=2
  wires:
  cfblk8/1 -> cfblk4/1
  cfblk6/1 -> cfblk3/1
  cfblk3/1 -> cfblk11/1
  cfblk5/1 -> cfblk6/1
  cfblk9/1 -> cfblk5/1
  cfblk1/1 -> cfblk6/2
  cfblk4/1 -> cfblk7/1
  cfblk10/1 -> cfblk2/1

== system sampleModel27/cfblk87/cfblk17/cfblk8/cfblk9 ==
  cfblk1 : Inport
  cfblk8 : Inport  Port=2
  cfblk9 : Inport  Port=3
  cfblk10 : Inport  Port=4
  cfblk11 : Inport  Port=5
  cfblk3 : simulink/Discrete/Transfer Fcn Real Zero  ZeroZ=0.75  ICPrevInput=0.0  DoSatur=off
      settings: SourceProductBaseCode=SL
  cfblk4 : Constant  Value=[237759127.475437]  SampleTime=1
  cfblk5 : Constant  Value=[794022935.961325]  SampleTime=1
  cfblk6 : Constant  Value=[-726030383.117919]  SampleTime=1
  cfblk7 : Constant  Value=[-904004578.852486]  SampleTime=1
  cfblk2 : Outport
  cfblk12 : Outport  Port=2
  cfblk13 : Outport  Port=3
  wires:
  cfblk11/1 -> cfblk2/1
  cfblk8/1 -> cfblk3/1
  cfblk4/1 -> cfblk13/1
  cfblk7/1 -> cfblk12/1

== system sampleModel27/cfblk87/cfblk17/cfblk9/cfblk10 ==
  cfblk1 : Inport
  cfblk8 : Inport  Port=2
  cfblk9 : Inport  Port=3
  cfblk10 : Inport  Port=4
  cfblk3 : simulink/Discrete/Tapped Delay  vinit=0.0  samptime=-1  NumDelays=1  DelayOrder=Oldest  includeCurrent=off
  cfblk4 : simulink/Discrete/Transfer Fcn Lead or Lag  PoleZ=0.95  ZeroZ=0.75  ICPrevOutput=0.0  ICPrevInput=0.0  DoSatur=off
      settings: SourceProductBaseCode=SL
  cfblk5 : Product  Inputs=*
  cfblk6 : DotProduct  InputSameDT=on  OutDataTypeStr=Inherit: Inherit via internal rule
  cfblk7 : Constant  Value=[794479508.873052]  SampleTime=1
  cfblk2 : Outport
  cfblk11 : Outport  Port=2
  wires:
  cfblk1/1 -> cfblk5/1
  cfblk6/1 -> cfblk2/1
  cfblk8/1 -> cfblk6/1
  cfblk3/1 -> cfblk6/2
  cfblk10/1 -> cfblk11/1
  cfblk7/1 -> cfblk4/1
  cfblk5/1 -> cfblk3/1

== system sampleModel27/cfblk93/cfblk11/cfblk14/cfblk8 ==
  cfblk1 : Inport
  cfblk6 : Inport  Port=2
  cfblk7 : Inport  Port=3
  cfblk8 : Inport  Port=4
  cfblk9 : Inport  Port=5
  cfblk3 : Constant  Value=[-496897468.126812]  SampleTime=1
  cfblk4 : Constant  Value=[846255544.534657]  SampleTime=1
  cfblk5 : Constant  Value=[-500624789.202451]  SampleTime=1
  cfblk2 : Outport
  wires:
  cfblk6/1 -> cfblk2/1

== system sampleModel27/cfblk93/cfblk11/cfblk18/cfblk10 ==
  cfblk1 : Inport
  cfblk8 : Inport  Port=2
  cfblk9 : Inport  Port=3
  cfblk10 : Inport  Port=4
  cfblk11 : Inport  Port=5
  cfblk12 : Inport  Port=6
  cfblk3 : pid_lib/PID Controller  Controller=PID  Form=Parallel  TimeDomain=Discrete-time  UseExternalTs=off  SampleTime=-1  IntegratorMethod=Forward Euler  FilterMethod=Forward Euler  ControllerParametersSource=internal  P=1  I=1  D=0  UseFilter=on  N=100  TunerSelectOption=Transfer Function Based (PID Tuner App)  InitialConditionSource=internal  InitialConditionForIntegrator=0  InitialConditionForFilter=0  DifferentiatorICPrevScaledInput=0  ExternalReset=none  TrackingMode=off  Kt=1  LimitOutput=off  SatLimitsSource=internal  UpperSaturationLimit=inf  LowerSaturationLimit=-inf  LinearizeAsGain=off  AntiWindupMode=none  Kb=1  POutMin=[]  POutMax=[]  IOutMin=[]  IOutMax=[]  DOutMin=[]  DOutMax=[]  NOutMin=[]  NOutMax=[]  SumOutMin=[]  SumOutMax=[]  SaturationOutMin=[]  SaturationOutMax=[]  PParamMin=[]  PParamMax=[]  IParamMin=[]  IParamMax=[]  DParamMin=[]  DParamMax=[]  NParamMin=[]  NParamMax=[]  KbParamMin=[]  KbParamMax=[]  KtParamMin=[]  KtParamMax=[]  KbOutMin=[]  KbOutMax=[]  KtOutMin=[]  KtOutMax=[]  IntegratorOutMin=[]  IntegratorOutMax=[]  FilterOutMin=[]  FilterOutMax=[]  SumI1OutMin=[]  SumI1OutMax=[]  SumI2OutMin=[]  SumI2OutMax=[]  SumI3OutMin=[]  SumI3OutMax=[]  SumI4OutMin=[]  SumI4OutMax=[]  SumDOutMin=[]  SumDOutMax=[]  DifferentiatorOutMin=[]  DifferentiatorOutMax=[]  FilterDiffOutCoefMin=[]  FilterDiffOutCoefMax=[]  ReciprocalOutMin=[]  ReciprocalOutMax=[]  SumDenOutMin=[]  SumDenOutMax=[]  SumNumOutMin=[]  SumNumOutMax=[]  DivideOutMin=[]  DivideOutMax=[]  UdiffTsProdOutMin=[]  UdiffTsProdOutMax=[]  NTsProdOutMin=[]  NTsProdOutMax=[]  UintegralTsProdOutMin=[]  UintegralTsProdOutMax=[]  UngainTsProdOutMin=[]  UngainTsProdOutMax=[]  IntegratorContinuousStateAttributes=''  IntegratorStateMustResolveToSignalObject=off  IntegratorRTWStateStorageClass=Auto  FilterContinuousStateAttributes=''  FilterStateMustResolveToSignalObject=off  FilterRTWStateStorageClass=Auto  ParallelPVariant=InternalParameters  IdealPVariant=Disabled  IVariant=InternalParameters  DVariant=InternalParameters  IntegratorVariant=Discrete  SatVariant=Disabled  AWVariant=Passthrough  PCopyVariant=Disabled  TRVariant=Disabled  FdbkBlocksVariant=Forward  IdealPFdbkVariant=Disabled  SatFdbkVariant=Disabled  DerivativeFilterVariant=ForwardEulerFilter  NVariant=InternalParameters  NCopyVariant=Disabled  FilterICVariant=InternalICsFilter  IntegratorICVariant=InternalICs  ExternalResetVariant=Disabled  TRSumVariant=Passthrough  SumFdbkVariant=Disabled  SumVariant=Sum_PID  TsampFilterVariant=InternalTs  TsampNgainVariant=Passthrough  TsampIntegralVariant=Passthrough  ExternalSaturationOutDataTypeStr=Inherit: Same as second input
  cfblk4 : Sum  Inputs=+-
  cfblk5 : Reshape
  cfblk6 : Constant  Value=[265653972.163588]  SampleTime=1
  cfblk7 : Constant  Value=[627876204.115601]  SampleTime=1
  cfblk2 : Outport
  wires:
  cfblk10/1 -> cfblk2/1
  cfblk11/1 -> cfblk5/1
  cfblk12/1 -> cfblk4/1
  cfblk7/1 -> cfblk4/2
  cfblk5/1 -> cfblk3/1

== system sampleModel27/cfblk93/cfblk11/cfblk19/cfblk8 ==
  cfblk1 : Inport
  cfblk7 : Inport  Port=2
  cfblk3 : simulink/Discrete/Transfer Fcn First Order  PoleZ=0.95  ICPrevOutput=0.0  DoSatur=off
  cfblk4 : Constant  Value=[740948994.862408]  SampleTime=1
  cfblk5 : Constant  Value=[-681786426.112416]  SampleTime=1
  cfblk6 : Constant  Value=[284838188.609533]  SampleTime=1
  cfblk2 : Outport
  cfblk8 : Outport  Port=2
  wires:
  cfblk6/1 -> cfblk2/1
  cfblk4/1 -> cfblk8/1
  cfblk5/1 -> cfblk3/1

== system sampleModel27/cfblk95/cfblk12/cfblk11/cfblk10 ==
  cfblk1 : Inport
  cfblk8 : Inport  Port=2
  cfblk9 : Inport  Port=3
  cfblk10 : Inport  Port=4
  cfblk3 : DiscreteTransferFcn
  cfblk4 : UnitDelay  SampleTime=-1  HasFrameUpgradeWarning=on
  cfblk5 : Constant  Value=[-525176114.723447]  SampleTime=1
  cfblk6 : Constant  Value=[-363794187.541583]  SampleTime=1
  cfblk7 : Constant  Value=[659275320.174151]  SampleTime=1
  cfblk2 : Outport
  wires:
  cfblk3/1 -> cfblk2/1
  cfblk8/1 -> cfblk4/1
  cfblk9/1 -> cfblk3/1

== system sampleModel27/cfblk95/cfblk12/cfblk11/cfblk11 ==
  cfblk1 : Inport
  cfblk16 : Inport  Port=2
  cfblk10 : Constant  Value=[470383047.367433]  SampleTime=1
  cfblk11 : Constant  Value=[-93063590.586734]  SampleTime=1
  cfblk12 : Constant  Value=[116917676.809431]  SampleTime=1
  cfblk13 : Constant  Value=[-247499056.572446]  SampleTime=1
  cfblk14 : Constant  Value=[-290528305.099033]  SampleTime=1
  cfblk15 : Constant  Value=[-113437488.241104]  SampleTime=1
  cfblk3 : Sqrt  SaturateOnIntegerOverflow=on
  cfblk4 : simulink/Math Operations/MinMax Running Resettable  Function=min  vinit=0.0
  cfblk5 : Math  Operator=10^u  SaturateOnIntegerOverflow=on
  cfblk6 : ComplexToRealImag
  cfblk7 : Constant  Value=[-169983489.236740]  SampleTime=1
  cfblk8 : Constant  Value=[-506163727.451602]  SampleTime=1
  cfblk9 : Constant  Value=[-86053256.839859]  SampleTime=1
  cfblk2 : Outport
  wires:
  cfblk5/1 -> cfblk2/1
  cfblk16/1 -> cfblk6/1
  cfblk8/1 -> cfblk4/1
  cfblk9/1 -> cfblk4/2
  cfblk7/1 -> cfblk3/1
  cfblk12/1 -> cfblk5/1
